simulink library "sensors_lib"  (Simulink 7.2)
settings: Solver=ode45  SolverMode=SingleTasking  StartTime=0.0  StopTime=10.0  RelTol=1e-3
libraries: sensors_T2_lib x1, sensors_T2_design_lib x1, simulink x1, sensor_failure_lib x1, sensors_lib x1
settings Model: Creator=amurch  LastModifiedBy=la1032aw

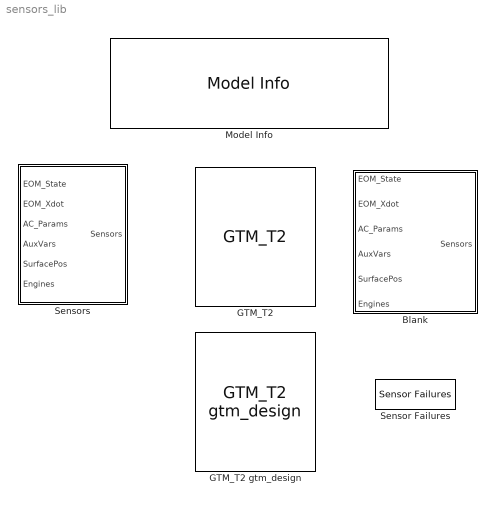
== system sensors_lib ==
  Blank : Subsystem
  GTM_T2 : sensors_T2_lib/GTM_T2  SystemSampleTime=-1
  GTM_T2 gtm_design : sensors_T2_design_lib/GTM_T2 gtm_design  SystemSampleTime=-1
  Model Info : simulink/Model-Wide Utilities/Model Info  SystemSampleTime=-1  InitialBlockCM=None  BlockCM=None  Frame=on  DisplayStringWithTags=|  HorizontalTextAlignment=Center  LeftAlignmentValue=0.5  SourceBlockDiagram=sensors_lib  TagMaxNumber=20
      | Sensor Model Library
      | %<ModelVersion>
      | Las modified by %<LastModifiedBy> on %<LastModificationDate>
  Sensor Failures : sensor_failure_lib/Sensor Failures  SystemSampleTime=-1
  Sensors : Subsystem  BlockChoice=Blank
      settings: TemplateBlock=self  MemberBlocks=Blank,GTM_T2,GTM_T2 gtm_design

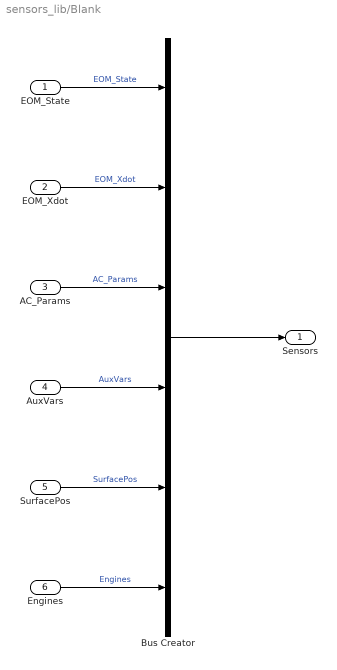
== system sensors_lib/Blank ==
  EOM_State : Inport  OutDataType=sfix(16)  OutScaling=2^0
  EOM_Xdot : Inport  Port=2  OutDataType=sfix(16)  OutScaling=2^0
  AC_Params : Inport  Port=3  OutDataType=sfix(16)  OutScaling=2^0
  AuxVars : Inport  Port=4  OutDataType=sfix(16)  OutScaling=2^0
  SurfacePos : Inport  Port=5  OutDataType=sfix(16)  OutScaling=2^0
  Engines : Inport  Port=6  OutDataType=sfix(16)  OutScaling=2^0
  Bus Creator : BusCreator  Inputs=6
  Sensors : Outport  OutDataType=sfix(16)  OutScaling=2^0
  wires:
  Bus Creator/1 -> Sensors/1
  EOM_State/1 -> Bus Creator/1  "EOM_State"
  EOM_Xdot/1 -> Bus Creator/2  "EOM_Xdot"
  AC_Params/1 -> Bus Creator/3  "AC_Params"
  AuxVars/1 -> Bus Creator/4  "AuxVars"
  SurfacePos/1 -> Bus Creator/5  "SurfacePos"
  Engines/1 -> Bus Creator/6  "Engines"

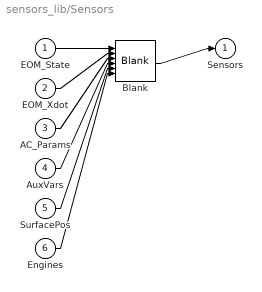
== system sensors_lib/Sensors ==
  EOM_State : Inport  OutDataType=sfix(16)  OutScaling=2^0
  EOM_Xdot : Inport  Port=2  OutDataType=sfix(16)  OutScaling=2^0
  AC_Params : Inport  Port=3  OutDataType=sfix(16)  OutScaling=2^0
  AuxVars : Inport  Port=4  OutDataType=sfix(16)  OutScaling=2^0
  SurfacePos : Inport  Port=5  OutDataType=sfix(16)  OutScaling=2^0
  Engines : Inport  Port=6  OutDataType=sfix(16)  OutScaling=2^0
  Blank : sensors_lib/Blank  SystemSampleTime=-1
  Sensors : Outport  OutDataType=sfix(16)  OutScaling=2^0
  wires:
  EOM_State/1 -> Blank/1
  EOM_Xdot/1 -> Blank/2
  AC_Params/1 -> Blank/3
  AuxVars/1 -> Blank/4
  SurfacePos/1 -> Blank/5
  Engines/1 -> Blank/6
  Blank/1 -> Sensors/1
